simulink subsystem "radio"  (R2023b)
settings: Solver=VariableStepAuto  StartTime=0.0  StopTime=10.0  RelTol=1e-3
undefined symbols (not defined in the file or in its folder): Environment, Radio
libraries: sensors_subsystems x9, simulink x3
settings Model: Creator=brent  LastModifiedBy=brent

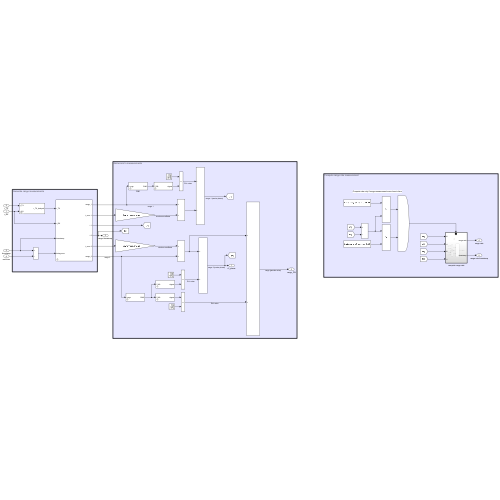
[thumbnail: Simulink's stored preview of the top-level diagram]
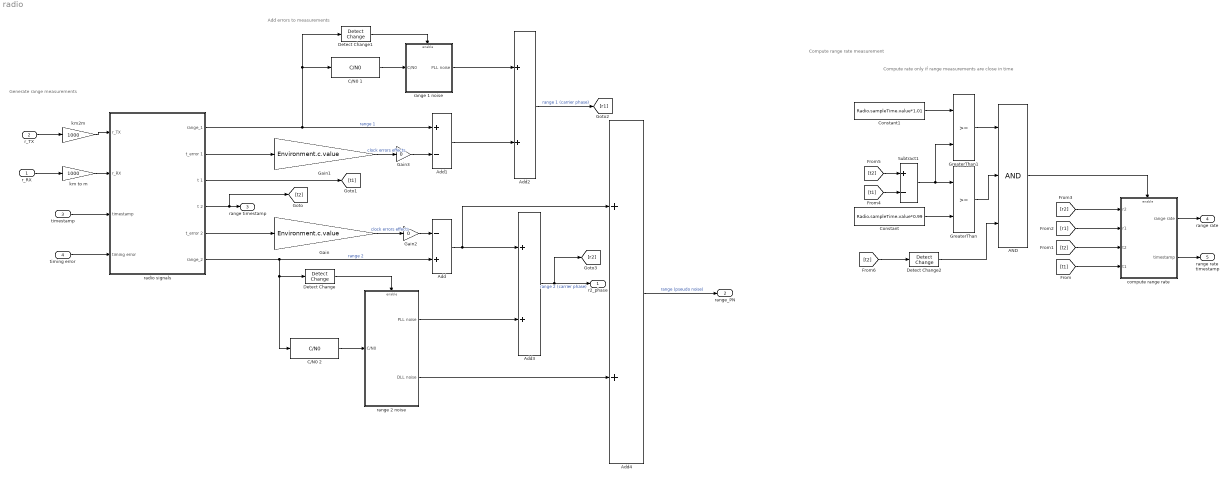
== system radio ==
  note: Compute range rate measurement
  note: Add errors to measurements
  note: Generate range measurements
  note: Compute rate only if range measurements are close in time
  r_RX : Inport
  r_TX : Inport  Port=2
  timestamp : Inport  Port=3
  timing error : Inport  Port=4
  AND : Logic  Inputs=3  IconShape=distinctive  AllPortsSameDT=off  OutDataTypeStr=boolean
  Add : Sum  Inputs=-+
  Add1 : Sum  Inputs=+-
  Add2 : Sum
  Add3 : Sum
  Add4 : Sum
  C/N0 1 : sensors_subsystems/C//N0  lambda=Radio.lambda.value  Pt=Radio.Tx.P.value  Gt=Radio.Tx.gain.value  Gr=Radio.Rx.gain.value  N0=Radio.N0.value  L_rx=Radio.Rx.losses.value
      settings: SourceProductName=Sensors library
  C/N0 2 : sensors_subsystems/C//N0  lambda=Radio.lambda.value  Pt=Radio.Tx.P.value  Gt=Radio.Tx.gain.value  Gr=Radio.Rx.gain.value  N0=Radio.N0.value  L_rx=Radio.Rx.losses.value
      settings: SourceProductName=Sensors library
  Constant : Constant  Value=Radio.sampleTime.value*0.99
  Constant1 : Constant  Value=Radio.sampleTime.value*1.01
  Detect Change : simulink/Logic and Bit Operations/Detect Change  vinit=0  OutDataTypeStr=boolean
  Detect Change1 : simulink/Logic and Bit Operations/Detect Change  vinit=0  OutDataTypeStr=boolean
  Detect Change2 : simulink/Logic and Bit Operations/Detect Change  vinit=0  OutDataTypeStr=boolean
  Gain : Gain  Gain=Environment.c.value
  Gain1 : Gain  Gain=Environment.c.value
  Gain2 : Gain  Gain=0
  Gain3 : Gain  Gain=0
  GreaterThan : RelationalOperator  OutDataTypeStr=boolean  RndMeth=Simplest  InputSameDT=off
  GreaterThan1 : RelationalOperator  OutDataTypeStr=boolean  RndMeth=Simplest  InputSameDT=off
  Subtract1 : Sum  Inputs=+-
  compute range rate : Subsystem
  km to m : Gain  Gain=1000
  "km2m " : Gain  Gain=1000
  radio signals : Subsystem  AncestorBlock=sensors_subsystems/radio signals  mask{light_speed=Environment.c.value, R_m=Environment.Moon.radius.value, sampleTime=Radio.sampleTime.value, delay=Radio.delay.value, pulseSamples=Radio.pulseSamples.value, pulseWidth=Radio.pulseWidth.value}
      mask prompts: light_speed "Speed of light"; R_m "Moon Radius"; sampleTime "Time between the two signals"; delay "Phase delay (samples)"; pulseSamples "Number of samples"; pulseWidth "Pulse width (samples)"
      mask DialogControl DescGroupVar Prompt: Range signals
      mask DialogControl DescTextVar Prompt: Simulate noise-free range signals
  range 1 noise : Subsystem  TreatAsAtomicUnit=on
  range 2 noise : Subsystem  TreatAsAtomicUnit=on
  r2_phase : Outport
  range_PN : Outport  Port=2
  "range timestamp " : Outport  Port=3
  range rate : Outport  Port=4
  range rate timestamp : Outport  Port=5
  wires:
  "km2m "/1 -> radio signals/1(r_TX)
  radio signals/6(range_2) -> Detect Change/1, C/N0 2/1, Add/2  "range 2"
  r_RX/1 -> km to m/1
  r_TX/1 -> "km2m "/1
  timestamp/1 -> radio signals/3(timestamp)
  timing error/1 -> radio signals/4(timing error)
  Add/1 -> Add4/1, Add3/1
  radio signals/1(range_1) -> Add1/1, C/N0 1/1, Detect Change1/1  "range 1"
  Add1/1 -> Add2/2
  Add2/1 -> [r1]  "range 1 (carrier phase)"
  Add3/1 -> [r2], r2_phase/1  "range 2 (carrier phase)"
  Add4/1 -> range_PN/1  "range (pseudo noise)"
  radio signals/2(t_error 1) -> Gain1/1
  radio signals/3(t 1) -> [t1]
  [r2] -> compute range rate/1(r2)
  [r1] -> compute range rate/2(r1)
  [t2] -> compute range rate/3(t2)
  [t1] -> compute range rate/4(t1)
  compute range rate/1(range rate) -> range rate/1
  [t1] -> Subtract1/2
  [t2] -> Subtract1/1
  Subtract1/1 -> GreaterThan1/2, GreaterThan/1
  Constant/1 -> GreaterThan/2
  Constant1/1 -> GreaterThan1/1
  GreaterThan/1 -> AND/2
  GreaterThan1/1 -> AND/1
  km to m/1 -> radio signals/2(r_RX)
  AND/1 -> compute range rate/Enable
  [t2] -> Detect Change2/1
  Detect Change2/1 -> AND/3
  Gain1/1 -> Gain3/1  "clock errors effects"
  Gain/1 -> Gain2/1  "clock errors effects"
  radio signals/4(t 2) -> [t2], "range timestamp "/1
  radio signals/5(t_error 2) -> Gain/1
  compute range rate/2(timestamp) -> range rate timestamp/1
  C/N0 2/1 -> range 2 noise/1(C/N0)
  range 2 noise/2(DLL noise) -> Add4/2
  range 2 noise/1(PLL noise) -> Add3/2
  Detect Change/1 -> range 2 noise/Enable
  C/N0 1/1 -> range 1 noise/1(C/N0)
  range 1 noise/1(PLL noise) -> Add2/1
  Detect Change1/1 -> range 1 noise/Enable
  Gain2/1 -> Add/1
  Gain3/1 -> Add1/2

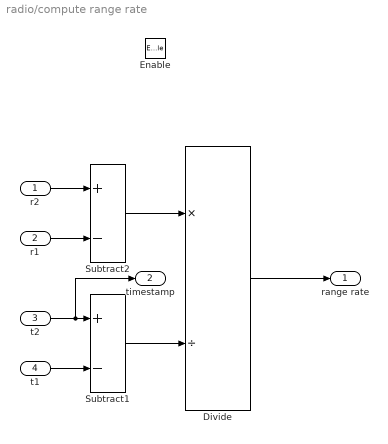
== system radio/compute range rate ==
  r2 : Inport
  r1 : Inport  Port=2
  t2 : Inport  Port=3
  t1 : Inport  Port=4
  Enable : EnablePort
  Divide : Product  Inputs=*/
  Subtract1 : Sum  Inputs=+-
  Subtract2 : Sum  Inputs=+-
  range rate : Outport
  timestamp : Outport  Port=2
  wires:
  r2/1 -> Subtract2/1
  Subtract1/1 -> Divide/2
  Divide/1 -> range rate/1
  Subtract2/1 -> Divide/1
  r1/1 -> Subtract2/2
  t2/1 -> timestamp/1, Subtract1/1
  t1/1 -> Subtract1/2

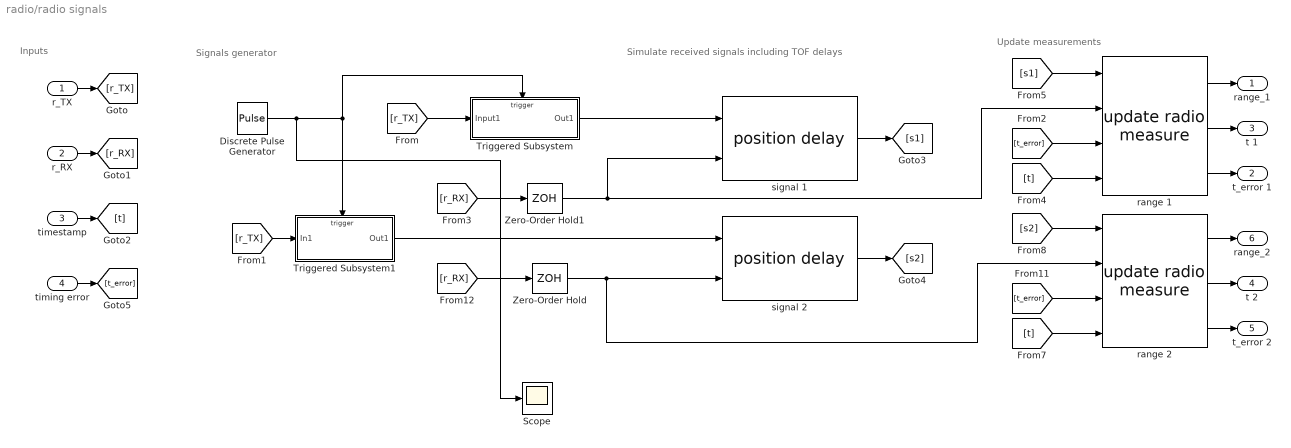
== system radio/radio signals ==
  note: Inputs
  note: Update measurements
  note: Simulate received signals including TOF delays
  note: Signals generator
  r_TX : Inport
  r_RX : Inport  Port=2
  timestamp : Inport  Port=3
  timing error : Inport  Port=4
  Discrete Pulse Generator : DiscretePulseGenerator  Period=pulseSamples  PulseWidth=pulseWidth  PhaseDelay=delay  SampleTime=sampleTime
  Scope : Scope
  Triggered Subsystem : Subsystem  TreatAsAtomicUnit=on
  Triggered Subsystem1 : Subsystem  TreatAsAtomicUnit=on
  Zero-Order Hold : ZeroOrderHold  SampleTime=-1
  Zero-Order Hold1 : ZeroOrderHold  SampleTime=-1
  range 1 : sensors_subsystems/update radio measure  R_m=R_m
      settings: SourceProductName=Sensors library
  range 2 : sensors_subsystems/update radio measure  R_m=R_m
      settings: SourceProductName=Sensors library
  signal 1 : sensors_subsystems/position delay  light_speed=light_speed
      settings: SourceProductName=Sensors library
  signal 2 : sensors_subsystems/position delay  light_speed=light_speed
      settings: SourceProductName=Sensors library
  range_1 : Outport
  t_error 1 : Outport  Port=2
  t 1 : Outport  Port=3
  t 2 : Outport  Port=4
  t_error 2 : Outport  Port=5
  range_2 : Outport  Port=6
  wires:
  Zero-Order Hold1/1 -> range 1/2, signal 1/2
  Zero-Order Hold/1 -> signal 2/2, range 2/2
  [t_error] -> range 2/3
  [t] -> range 2/4
  range 2/2 -> t 2/1
  range 2/3 -> t_error 2/1
  range 2/1 -> range_2/1
  [t_error] -> range 1/3
  timing error/1 -> [t_error]
  [t] -> range 1/4
  range 1/3 -> t_error 1/1
  Triggered Subsystem1/1(Out1) -> signal 2/1
  Triggered Subsystem/1(Out1) -> signal 1/1
  [r_TX] -> Triggered Subsystem/1(Input1)
  Discrete Pulse Generator/1 -> Triggered Subsystem1/Trigger, Triggered Subsystem/Trigger, Scope/1
  r_TX/1 -> [r_TX]
  r_RX/1 -> [r_RX]
  [r_TX] -> Triggered Subsystem1/1(In1)
  timestamp/1 -> [t]
  signal 1/1 -> [s1]
  signal 2/1 -> [s2]
  [s1] -> range 1/1
  [r_RX] -> Zero-Order Hold1/1
  [s2] -> range 2/1
  [r_RX] -> Zero-Order Hold/1
  range 1/2 -> t 1/1
  range 1/1 -> range_1/1

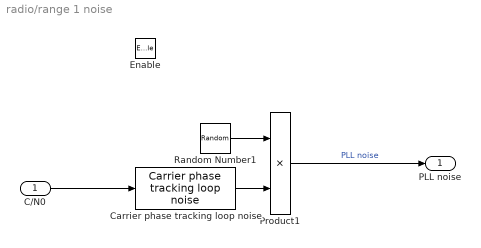
== system radio/range 1 noise ==
  C/N0 : Inport
  Enable : EnablePort
  Carrier phase tracking loop noise : sensors_subsystems/Carrier phase tracking loop noise  Bn=Radio.Phase.Bn.value  T=Radio.Phase.T.value  lambda=Radio.lambda.value
      settings: SourceProductName=Sensors library
  Product1 : Product
  Random Number1 : RandomNumber  Seed=abs(round(randn(1)*10^4))
  PLL noise : Outport
  wires:
  Product1/1 -> PLL noise/1  "PLL noise"
  Carrier phase tracking loop noise/1 -> Product1/2
  C/N0/1 -> Carrier phase tracking loop noise/1
  Random Number1/1 -> Product1/1

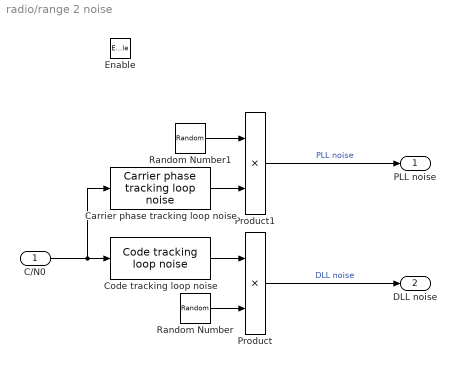
== system radio/range 2 noise ==
  C/N0 : Inport
  Enable : EnablePort
  Carrier phase tracking loop noise : sensors_subsystems/Carrier phase tracking loop noise  Bn=Radio.Phase.Bn.value  T=Radio.Phase.T.value  lambda=Radio.lambda.value
      settings: SourceProductName=Sensors library
  Code tracking loop noise : sensors_subsystems/Code tracking loop noise  Bn=Radio.PN.Bn.value  D=Radio.PN.D.value  T=Radio.PN.T.value  Tc=Radio.PN.Tc.value  Bfe=Radio.PN.Bfe.value  lambda=Radio.PN.lambda_c.value
      settings: SourceProductName=Sensors library
  Product : Product
  Product1 : Product
  Random Number : RandomNumber  Seed=abs(round(randn(1)*10^4))
  Random Number1 : RandomNumber  Seed=abs(round(randn(1)*10^4))
  PLL noise : Outport
  DLL noise : Outport  Port=2
  wires:
  Random Number1/1 -> Product1/1
  C/N0/1 -> Carrier phase tracking loop noise/1, Code tracking loop noise/1
  Carrier phase tracking loop noise/1 -> Product1/2
  Product1/1 -> PLL noise/1  "PLL noise"
  Code tracking loop noise/1 -> Product/1
  Random Number/1 -> Product/2
  Product/1 -> DLL noise/1  "DLL noise"

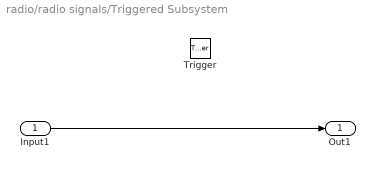
== system radio/radio signals/Triggered Subsystem ==
  Input1 : Inport
  Trigger : TriggerPort  VariantControl=(inherit)
  Out1 : Outport
  wires:
  Input1/1 -> Out1/1

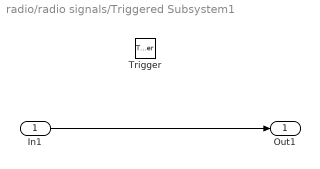
== system radio/radio signals/Triggered Subsystem1 ==
  In1 : Inport
  Trigger : TriggerPort  TriggerType=falling  VariantControl=(inherit)
  Out1 : Outport
  wires:
  In1/1 -> Out1/1
